simulink model "test_diode"  (R2021a)
settings: Solver=VariableStepAuto  StartTime=0.0  StopTime=0.1  RelTol=1e-3
libraries: spsDiodeLib x6, spsThreePhaseSeriesRLCBranchLib x2, spsMultimeterLib x2, spsSeriesRLCBranchLib x2, spsThreePhaseSourceLib x1, spspowerguiLib x1
settings Model: Creator=viliv  LastModifiedBy=viliv

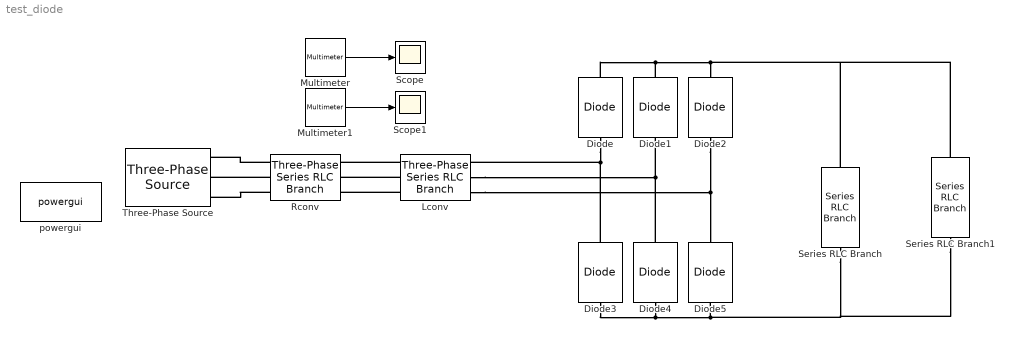
== system test_diode ==
  Diode{,1..5} (6 alike) : spsDiodeLib/Diode  Ron=1e-8  Lon=0  Vf=0.8  IC=0  UseSnubber=0  Rs=1e6  Cs=250e-12  Measurements=off
  Lconv : spsThreePhaseSeriesRLCBranchLib/Three-Phase Series RLC Branch  LConnTagsString=A|B|C  RConnTagsString=A|B|C  BranchType=L  Resistance=1  Inductance=100e-6  Capacitance=1e-6  Measurements=Branch currents
  Multimeter : spsMultimeterLib/Multimeter  PhasorSimulation=off  OutputType=Complex  sel=1  L=10  Gain=1  yselected={'Ub: Series RLC Branch'};  PSBOutputType=1  PSBequivalent=0  AxesSetting=[0,0.1,-100,100]  Display=0  SavedBlockNames=-11
  Multimeter1 : spsMultimeterLib/Multimeter  PhasorSimulation=off  OutputType=Complex  sel=[5 6 7]  L=10  Gain=[1 1 1]  yselected={'Ib1: Lconv','Ib2: Lconv','Ib3: Lconv'};  PSBOutputType=1  PSBequivalent=0  AxesSetting=[0,0.1,-100,100]  Display=0  SavedBlockNames=-11
  Rconv : spsThreePhaseSeriesRLCBranchLib/Three-Phase Series RLC Branch  LConnTagsString=A|B|C  RConnTagsString=A|B|C  BranchType=R  Resistance=1e-3  Inductance=0.1  Capacitance=1e-6  Measurements=Branch voltages and currents
  Scope : Scope
  Scope1 : Scope
  Series RLC Branch : spsSeriesRLCBranchLib/Series RLC Branch  LConnTagsString=__new0  RConnTagsString=__new0  BranchType=RC  Resistance=1e-3  Inductance=1e-3  SetiL0=off  InitialCurrent=0  Capacitance=10e-3  Setx0=off  InitialVoltage=0  Measurements=Branch voltage
  Series RLC Branch1 : spsSeriesRLCBranchLib/Series RLC Branch  LConnTagsString=__new0  RConnTagsString=__new0  BranchType=R  Resistance=1  Inductance=1e-3  SetiL0=off  InitialCurrent=0  Capacitance=0.05  Setx0=off  InitialVoltage=0  Measurements=None
  Three-Phase Source : spsThreePhaseSourceLib/Three-Phase Source  InternalConnection=Y  VoltagePhases=off  Voltage=400 * sqrt(3) / sqrt(2)  PhaseAngle=180  Voltage_phases=[25e3 25e3 25e3]/sqrt(3)  PhaseAngles_phases=[0 -120 +120]  Frequency=50  NonIdealSource=off  SpecifyImpedance=off  Resistance=0.8929  Inductance=16.58e-3  ShortCircuitLevel=100e6  BaseVoltage=25e3  XRratio=7  BusType=swing  Pref=10e3  Qref=0  Prefabc=[10e3, 10e3, 10e3]  Qrefabc=[0, 0, 0]  Qmin=-inf  Qmax=inf
  powergui : spspowerguiLib/powergui  Priority=1  SimulationMode=Discrete  SampleTime=10e-6  frequency=60  Iterations=50  frequencyindice=50  Pbase=100e6  ErrMax=1e-4  UnitsV=kV  UnitsW=MW  buscounter=0  FunctionMessages=off  echomessages=off  EnableUseOfTLC=off  CurrentSourceSwitches=off  DisableSnubberDevices=off  DisableRonSwitches=off  DisableVfSwitches=off  DisplayEquations=off  AutomaticDiscreteSolvers=off  SolverType=Tustin  Interpol=off  ExternalGateDelay=off  methode=off  Ts=100  x0status=zero  SPID=on  SwTol=0  HookPort=off  NonlinearTolerance=1e-4  nMaxIteration=100  ContinueOnMaxIteration=off  RestoreLinks=warning  ResistiveCurrentMeasurement=off  Frange=[0:2:500]  Ylog=off  Xlog=on  ShowGrid=off  save=off  variable=ZData  structure=0  ZoomFFT=off  StartTime=0.0  cycles=1  DisplayStyle=1  fundamental=60  FreqAxis=off  MaxFrequency=1000  frequencyindicesteady=1  RmsSteady=1  display=off
  wires:
  Multimeter/1 -> Scope/1
  Multimeter1/1 -> Scope1/1
  connections:
  Rconv/LConn2 -- Three-Phase Source/RConn2
  Rconv/LConn1 -- Three-Phase Source/RConn1
  Rconv/LConn3 -- Three-Phase Source/RConn3
  Lconv/LConn1 -- Rconv/RConn1
  Lconv/LConn2 -- Rconv/RConn2
  Lconv/LConn3 -- Rconv/RConn3
  Lconv/RConn2 -- Diode4/RConn1 -- Diode1/LConn1
  Diode/LConn1 -- Diode3/RConn1 -- Lconv/RConn1
  Lconv/RConn3 -- Diode5/RConn1 -- Diode2/LConn1
  Diode/RConn1 -- Diode1/RConn1 -- Series RLC Branch1/LConn1 -- Series RLC Branch/LConn1 -- Diode2/RConn1
  Diode3/LConn1 -- Diode4/LConn1 -- Series RLC Branch1/RConn1 -- Series RLC Branch/RConn1 -- Diode5/LConn1
